simulink model "ex2"  (R2024b)
settings: Solver=VariableStepAuto  StartTime=0.0  StopTime=10.0  RelTol=1e-3
settings Model: Creator=matei  LastModifiedBy=matei

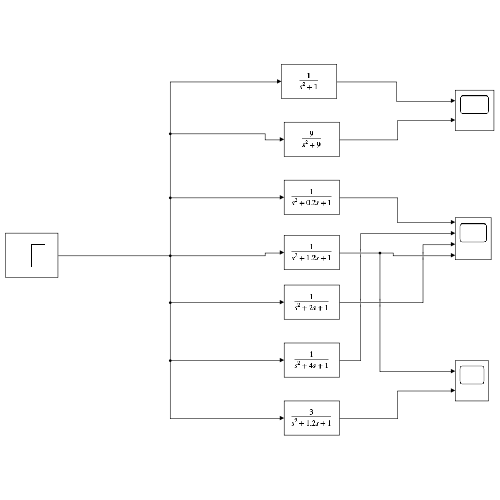
[thumbnail: Simulink's stored preview of the top-level diagram]
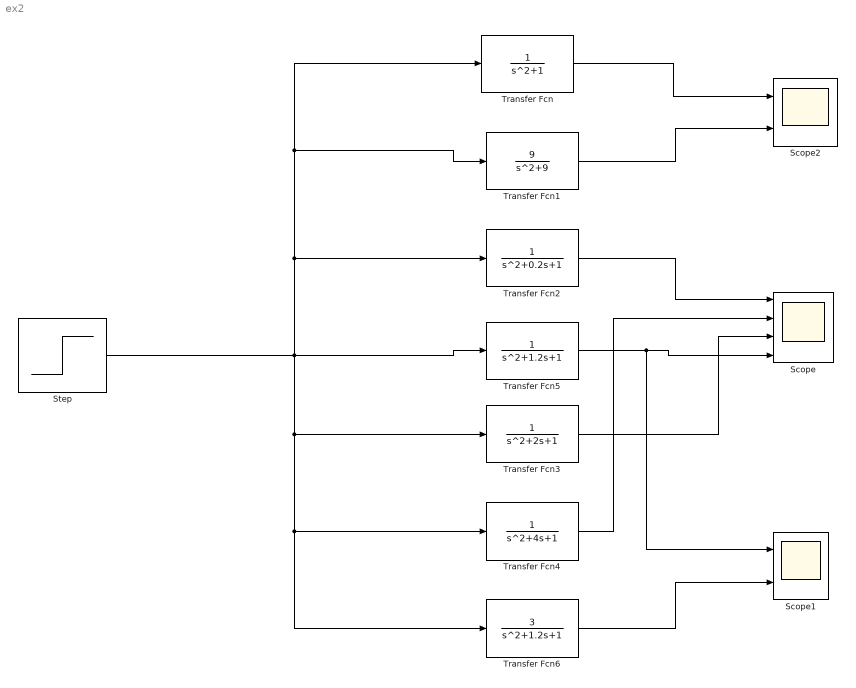
== system ex2 ==
  Scope : Scope  NumInputPorts=4
  Scope1 : Scope  NumInputPorts=2
  Scope2 : Scope  NumInputPorts=2
  Step : Step  SampleTime=0
  Transfer Fcn : TransferFcn  Denominator=[1 0 1]
  Transfer Fcn1 : TransferFcn  Numerator=[9]  Denominator=[1 0 9]
  Transfer Fcn2 : TransferFcn  Denominator=[1 0.2 1]
  Transfer Fcn3 : TransferFcn
  Transfer Fcn4 : TransferFcn  Denominator=[1 4 1]
  Transfer Fcn5 : TransferFcn  Denominator=[1 1.2 1]
  Transfer Fcn6 : TransferFcn  Numerator=[3]  Denominator=[1 1.2 1]
  wires:
  Step/1 -> Transfer Fcn3/1, Transfer Fcn4/1, Transfer Fcn6/1, Transfer Fcn5/1, Transfer Fcn2/1, Transfer Fcn1/1, Transfer Fcn/1
  Transfer Fcn5/1 -> Scope1/1, Scope/4
  Transfer Fcn2/1 -> Scope/1
  Transfer Fcn3/1 -> Scope/3
  Transfer Fcn4/1 -> Scope/2
  Transfer Fcn6/1 -> Scope1/2
  Transfer Fcn1/1 -> Scope2/2
  Transfer Fcn/1 -> Scope2/1
